simulink model "charge_and_discharge"  (R2021b)
settings: Solver=VariableStepAuto  StartTime=0.0  StopTime=1  RelTol=1e-3
undefined symbols (not defined in the file): Ion, Lithium
libraries: spsCurrentMeasurementLib x2, spsMosfetLib x2, spsBatteryLib x1, spsDCVoltageSourceLib x1, spsSeriesRLCBranchLib x1, spspowerguiLib x1
settings Model: Creator=eee  LastModifiedBy=eee

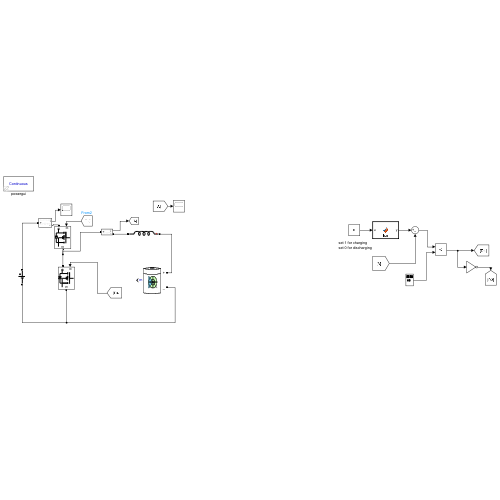
[thumbnail: Simulink's stored preview of the top-level diagram]
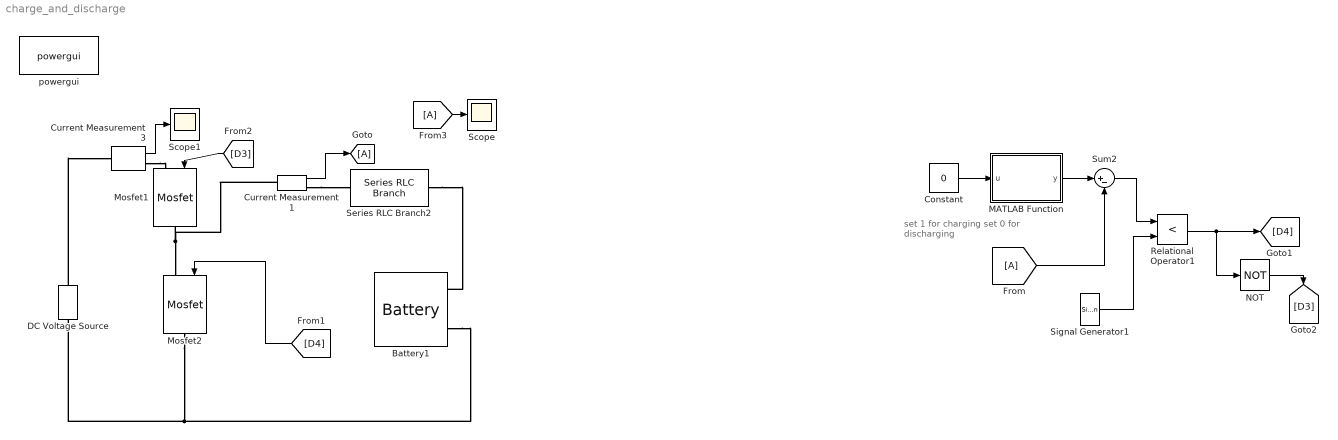
== system charge_and_discharge ==
  note: set 1 for charging
      | set 0 for discharging
  Battery1 : spsBatteryLib/Battery  BatType=Lithium-Ion  ShowTempParam=off  ThermalPreset=no  ShowAgeParam=off  NomV=192  NomQ=100  SOC=50  Batt_Tr=30  PresetModel=on  MaxQ=100  MinV=144  FullV=223.4855  Dis_rate=43.4783  R=0.0192  Normal_OP=90.4348  expZone="[207.4341      4.913043]"  current=[6.5 13 32.5]  Units=Time  Tci=20  NomT=20  T2=-30  MaxQ2=4.8  FullV2=7.1  Normal_OP2=5.655  expZone2="[6.58           1]"  Rca=0.6  ti=2000  Dp=0  Neq0=0  Tsim=1e6  Ta1=25  Qeol=5.4*0.9  Reol=0.013333*1.2  Char_age=[2.3478, 3]  Dis_age=[2.3478, 10]  N1=1500  N2=10500  N3=1000  N4=1400  Ta2=45  N5=950
  Constant : Constant  Value=0
  Current Measurement1 : spsCurrentMeasurementLib/Current Measurement  PhasorSimulation=off  OutputType=Complex  PSBequivalent=0
  Current Measurement3 : spsCurrentMeasurementLib/Current Measurement  PhasorSimulation=off  OutputType=Complex  PSBequivalent=0
  DC Voltage Source : spsDCVoltageSourceLib/DC Voltage Source  Amplitude=350  Measurements=None
  MATLAB Function : MATLAB Function  TreatAsAtomicUnit=on
  Mosfet1 : spsMosfetLib/Mosfet  Ron=0.1  Lon=0  Rd=0.01  Vfd=0  IC=0  Rs=1e5  Cs=inf  Measurements=off
  Mosfet2 : spsMosfetLib/Mosfet  Ron=0.1  Lon=0  Rd=0.01  Vfd=0  IC=0  Rs=1e5  Cs=inf  Measurements=off
  NOT : Logic  Operator=NOT  IconShape=distinctive  AllPortsSameDT=off  OutDataTypeStr=boolean
  Relational Operator1 : RelationalOperator  Operator=<  OutDataTypeStr=boolean  RndMeth=Simplest
  Scope : Scope
  Scope1 : Scope
  Series RLC Branch2 : spsSeriesRLCBranchLib/Series RLC Branch  LConnTagsString=__new0  RConnTagsString=__new0  BranchType=L  Resistance=1  Inductance=5*1e-3  SetiL0=off  InitialCurrent=0  Capacitance=1e-6  Setx0=off  InitialVoltage=0  Measurements=None
  Signal Generator1 : SignalGenerator  WaveForm=sawtooth  Frequency=20000
  Sum2 : Sum  Inputs=|+-
  powergui : spspowerguiLib/powergui  Priority=1  SimulationMode=Continuous  SampleTime=50e-6  frequency=60  Iterations=50  frequencyindice=0  Pbase=100e6  ErrMax=1e-4  UnitsV=kV  UnitsW=MW  buscounter=0  FunctionMessages=off  echomessages=off  EnableUseOfTLC=off  CurrentSourceSwitches=off  DisableSnubberDevices=off  DisableRonSwitches=off  DisableVfSwitches=off  DisplayEquations=off  AutomaticDiscreteSolvers=off  SolverType=Tustin/Backward Euler (TBE)  Interpol=off  ExternalGateDelay=off  methode=off  Ts=100  x0status=blocks  SPID=on  SwTol=0  HookPort=off  NonlinearTolerance=1e-4  nMaxIteration=100  ContinueOnMaxIteration=off  RestoreLinks=warning  ResistiveCurrentMeasurement=off  Frange=[0:2:500]  Ylog=off  Xlog=on  ShowGrid=off  save=off  variable=ZData  structure=0  ZoomFFT=off  StartTime=0.0  cycles=1  DisplayStyle=1  fundamental=60  FreqAxis=off  MaxFrequency=1000  frequencyindicesteady=1  RmsSteady=1  display=off
  wires:
  [D4] -> Mosfet2/1
  Constant/1 -> MATLAB Function/1(u)
  Relational Operator1/1 -> NOT/1, [D4]
  Sum2/1 -> Relational Operator1/1
  Current Measurement3/1 -> Scope1/1
  Current Measurement1/1 -> [A]
  Signal Generator1/1 -> Relational Operator1/2
  MATLAB Function/1(y) -> Sum2/1
  [A] -> Sum2/2
  NOT/1 -> [D3]
  [D3] -> Mosfet1/1
  [A] -> Scope/1
  connections:
  Battery1/LConn2 -- Mosfet2/RConn1 -- DC Voltage Source/LConn1
  Mosfet1/RConn1 -- Mosfet2/LConn1 -- Current Measurement1/LConn1
  Series RLC Branch2/LConn1 -- Battery1/LConn1
  DC Voltage Source/RConn1 -- Current Measurement3/LConn1
  Current Measurement3/RConn1 -- Mosfet1/LConn1
  Current Measurement1/RConn1 -- Series RLC Branch2/RConn1

== matlab function charge_and_discharge/MATLAB Function ==
  data: u input; y output
function y = fcn(u)
if(u==1)
    y=15;
else
    y=-15;
end
